simulink library "lib_Actuators"  (R2017a)
settings: Solver=VariableStepAuto  StartTime=0.0  StopTime=10.0  RelTol=1e-3
settings Model: Creator=Di Russo  LastModifiedBy=Vraj M

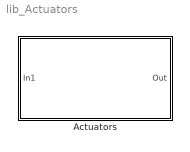
== system lib_Actuators ==
  Actuators : Subsystem

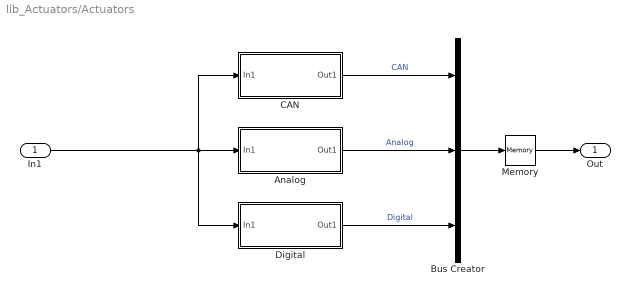
== system lib_Actuators/Actuators ==
  In1 : Inport
  Analog : Subsystem
  Bus Creator : BusCreator  Inputs=3
  CAN : Subsystem
  Digital : Subsystem
  Memory : Memory  InheritSampleTime=on
  Out : Outport
  wires:
  Memory/1 -> Out/1
  Analog/1(Out1) -> Bus Creator/2  "Analog"
  CAN/1(Out1) -> Bus Creator/1  "CAN"
  Digital/1(Out1) -> Bus Creator/3  "Digital"
  Bus Creator/1 -> Memory/1
  In1/1 -> Digital/1(In1), Analog/1(In1), CAN/1(In1)

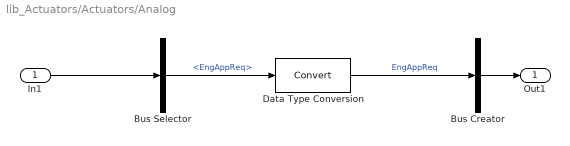
== system lib_Actuators/Actuators/Analog ==
  In1 : Inport
  Bus Creator : BusCreator  Inputs=1
  Bus Selector : BusSelector  OutputSignals=Controls.EngAppReq
  Data Type Conversion : DataTypeConversion
  Out1 : Outport
  wires:
  Data Type Conversion/1 -> Bus Creator/1  "EngAppReq"
  Bus Selector/1 -> Data Type Conversion/1  "<EngAppReq>"
  Bus Creator/1 -> Out1/1
  In1/1 -> Bus Selector/1

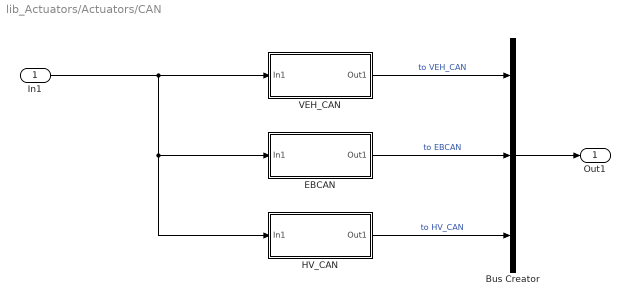
== system lib_Actuators/Actuators/CAN ==
  In1 : Inport
  Bus Creator : BusCreator  Inputs=3
  EBCAN : Subsystem
  HV_CAN : Subsystem
  VEH_CAN : Subsystem
  Out1 : Outport
  wires:
  In1/1 -> VEH_CAN/1(In1), EBCAN/1(In1), HV_CAN/1(In1)
  Bus Creator/1 -> Out1/1
  HV_CAN/1(Out1) -> Bus Creator/3  "to HV_CAN"
  EBCAN/1(Out1) -> Bus Creator/2  "to EBCAN"
  VEH_CAN/1(Out1) -> Bus Creator/1  "to VEH_CAN"

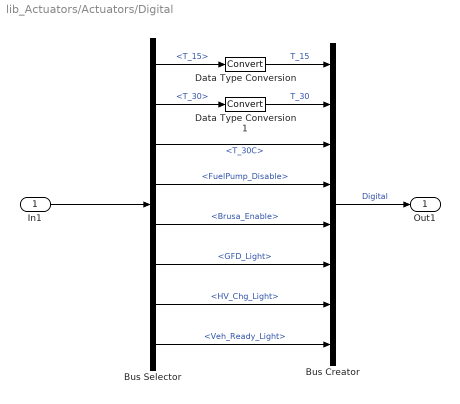
== system lib_Actuators/Actuators/Digital ==
  In1 : Inport
  Bus Creator : BusCreator  Inputs=8
  Bus Selector : BusSelector  OutputSignals=BMS_Digital.T_15,BMS_Digital.T_30,BMS_Digital.T_30C,Fuel_Pump_Control.Pump_Commands.FuelPump_Disable,OBC_Digital.Brusa_Enable,Axiomatic_CAN.GFD_Light,Axiomatic_CAN.HV_Chg_Light,Axiomatic_CAN.Veh_Ready_Light
  Data Type Conversion : DataTypeConversion
  Data Type Conversion1 : DataTypeConversion
  Out1 : Outport
  wires:
  Data Type Conversion1/1 -> Bus Creator/2  "T_30"
  Data Type Conversion/1 -> Bus Creator/1  "T_15"
  Bus Selector/8 -> Bus Creator/8  "<Veh_Ready_Light>"
  Bus Selector/7 -> Bus Creator/7  "<HV_Chg_Light>"
  Bus Selector/6 -> Bus Creator/6  "<GFD_Light>"
  Bus Selector/5 -> Bus Creator/5  "<Brusa_Enable>"
  Bus Selector/1 -> Data Type Conversion/1  "<T_15>"
  Bus Selector/2 -> Data Type Conversion1/1  "<T_30>"
  Bus Selector/3 -> Bus Creator/3  "<T_30C>"
  Bus Selector/4 -> Bus Creator/4  "<FuelPump_Disable>"
  Bus Creator/1 -> Out1/1  "Digital"
  In1/1 -> Bus Selector/1

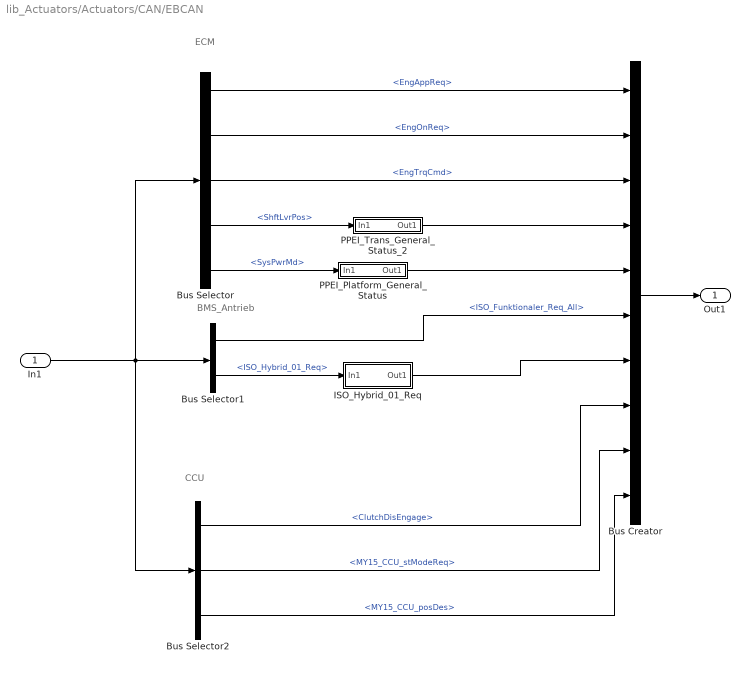
== system lib_Actuators/Actuators/CAN/EBCAN ==
  note: CCU
  note: ECM
  note: BMS_Antrieb
  In1 : Inport
  Bus Creator : BusCreator  Inputs=10
  Bus Selector : BusSelector  OutputSignals=Controls.EngAppReq,Controls.EngOnReq,Controls.EngTrqCmd,Controls.ShftLvrPos,Controls.SysPwrMd
  Bus Selector1 : BusSelector  OutputSignals=BMS_CAN.ISO_Funktionaler_Req_All,BMS_CAN.ISO_Hybrid_01_Req
  Bus Selector2 : BusSelector  OutputSignals=Controls.ClutchDisEngage,CCU_CAN.MY15_CCU_stModeReq,CCU_CAN.MY15_CCU_posDes
  ISO_Hybrid_01_Req : Subsystem
  PPEI_Platform_General_Status : Subsystem
  PPEI_Trans_General_Status_2 : Subsystem
  Out1 : Outport
  wires:
  Bus Selector2/1 -> Bus Creator/8  "<ClutchDisEngage>"
  Bus Selector2/3 -> Bus Creator/10  "<MY15_CCU_posDes>"
  Bus Selector2/2 -> Bus Creator/9  "<MY15_CCU_stModeReq>"
  In1/1 -> Bus Selector1/1, Bus Selector2/1, Bus Selector/1
  Bus Selector1/2 -> ISO_Hybrid_01_Req/1(In1)  "<ISO_Hybrid_01_Req>"
  ISO_Hybrid_01_Req/1(Out1) -> Bus Creator/7
  Bus Selector1/1 -> Bus Creator/6  "<ISO_Funktionaler_Req_All>"
  Bus Selector/1 -> Bus Creator/1  "<EngAppReq>"
  Bus Selector/2 -> Bus Creator/2  "<EngOnReq>"
  Bus Selector/3 -> Bus Creator/3  "<EngTrqCmd>"
  PPEI_Trans_General_Status_2/1(Out1) -> Bus Creator/4
  Bus Selector/5 -> PPEI_Platform_General_Status/1(In1)  "<SysPwrMd>"
  Bus Selector/4 -> PPEI_Trans_General_Status_2/1(In1)  "<ShftLvrPos>"
  PPEI_Platform_General_Status/1(Out1) -> Bus Creator/5
  Bus Creator/1 -> Out1/1

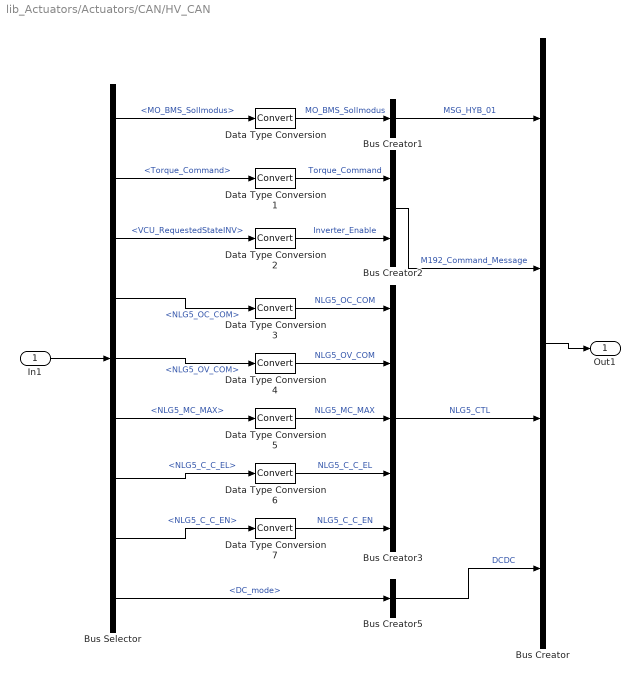
== system lib_Actuators/Actuators/CAN/HV_CAN ==
  In1 : Inport
  Bus Creator : BusCreator  Inputs=4
  Bus Creator1 : BusCreator  Inputs=1
  Bus Creator2 : BusCreator  Inputs=2
  Bus Creator3 : BusCreator  Inputs=5
  Bus Creator5 : BusCreator  Inputs=1
  Bus Selector : BusSelector  OutputSignals=BMS_CAN.MSG_HYB_01.MO_BMS_Sollmodus,Controls.Torque_Command,MCU_CAN.MCU_CAN.VCU_RequestedStateINV,OBC_CAN.NLG5_OC_COM,OBC_CAN.NLG5_OV_COM,OBC_CAN.NLG5_MC_MAX,OBC_CAN.NLG5_C_C_EL,OBC_CAN.NLG5_C_C_EN,MCU_CAN.DCDC_Out.DC_mode
  Data Type Conversion{,1..7} (8 alike) : DataTypeConversion
  Out1 : Outport
  wires:
  Bus Creator5/1 -> Bus Creator/4  "DCDC"
  Bus Selector/9 -> Bus Creator5/1  "<DC_mode>"
  Data Type Conversion7/1 -> Bus Creator3/5  "NLG5_C_C_EN"
  Data Type Conversion6/1 -> Bus Creator3/4  "NLG5_C_C_EL"
  Data Type Conversion5/1 -> Bus Creator3/3  "NLG5_MC_MAX"
  Data Type Conversion4/1 -> Bus Creator3/2  "NLG5_OV_COM"
  Data Type Conversion3/1 -> Bus Creator3/1  "NLG5_OC_COM"
  Bus Creator3/1 -> Bus Creator/3  "NLG5_CTL"
  Data Type Conversion2/1 -> Bus Creator2/2  "Inverter_Enable"
  Data Type Conversion1/1 -> Bus Creator2/1  "Torque_Command"
  Bus Selector/8 -> Data Type Conversion7/1  "<NLG5_C_C_EN>"
  Bus Selector/7 -> Data Type Conversion6/1  "<NLG5_C_C_EL>"
  Bus Selector/6 -> Data Type Conversion5/1  "<NLG5_MC_MAX>"
  Bus Selector/5 -> Data Type Conversion4/1  "<NLG5_OV_COM>"
  Bus Selector/4 -> Data Type Conversion3/1  "<NLG5_OC_COM>"
  Bus Creator2/1 -> Bus Creator/2  "M192_Command_Message"
  Bus Selector/3 -> Data Type Conversion2/1  "<VCU_RequestedStateINV>"
  Bus Selector/2 -> Data Type Conversion1/1  "<Torque_Command>"
  Bus Creator1/1 -> Bus Creator/1  "MSG_HYB_01"
  Data Type Conversion/1 -> Bus Creator1/1  "MO_BMS_Sollmodus"
  Bus Selector/1 -> Data Type Conversion/1  "<MO_BMS_Sollmodus>"
  In1/1 -> Bus Selector/1
  Bus Creator/1 -> Out1/1

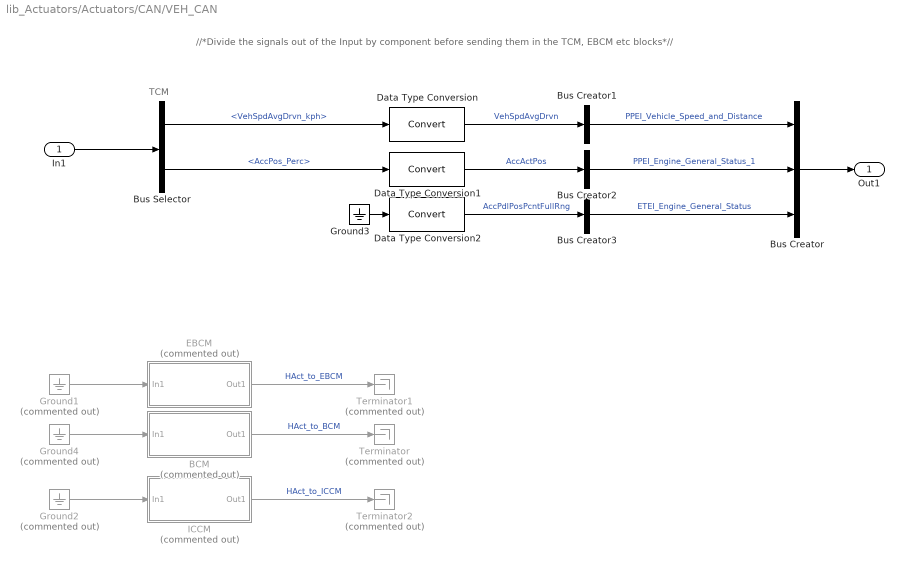
== system lib_Actuators/Actuators/CAN/VEH_CAN ==
  note: //*Divide the signals out of the Input by component before sending them in the TCM, EBCM etc blocks*//
  note: TCM
  In1 : Inport
  BCM : Subsystem  Commented=on
  Bus Creator : BusCreator  Inputs=3
  Bus Creator1 : BusCreator  Inputs=1
  Bus Creator2 : BusCreator  Inputs=1
  Bus Creator3 : BusCreator  Inputs=1
  Bus Selector : BusSelector  OutputSignals=Controls.VehSpdAvgDrvn_kph,Controls.AccPos_Perc
  Data Type Conversion : DataTypeConversion
  Data Type Conversion1 : DataTypeConversion
  Data Type Conversion2 : DataTypeConversion
  EBCM : Subsystem  Commented=on
  Ground1 : Ground  Commented=on
  Ground2 : Ground  Commented=on
  Ground3 : Ground
  Ground4 : Ground  Commented=on
  ICCM : Subsystem  Commented=on
  Terminator : Terminator  Commented=on
  Terminator1 : Terminator  Commented=on
  Terminator2 : Terminator  Commented=on
  Out1 : Outport
  wires:
  Ground4/1 -> BCM/1(In1)
  Ground3/1 -> Data Type Conversion2/1
  Data Type Conversion2/1 -> Bus Creator3/1  "AccPdlPosPcntFullRng"
  Bus Creator3/1 -> Bus Creator/3  "ETEI_Engine_General_Status"
  Bus Creator2/1 -> Bus Creator/2  "PPEI_Engine_General_Status_1"
  Data Type Conversion1/1 -> Bus Creator2/1  "AccActPos"
  Bus Creator1/1 -> Bus Creator/1  "PPEI_Vehicle_Speed_and_Distance"
  In1/1 -> Bus Selector/1
  Bus Selector/1 -> Data Type Conversion/1  "<VehSpdAvgDrvn_kph>"
  Bus Selector/2 -> Data Type Conversion1/1  "<AccPos_Perc>"
  Ground2/1 -> ICCM/1(In1)
  Ground1/1 -> EBCM/1(In1)
  Bus Creator/1 -> Out1/1
  Data Type Conversion/1 -> Bus Creator1/1  "VehSpdAvgDrvn"
  EBCM/1(Out1) -> Terminator1/1  "HAct_to_EBCM"
  BCM/1(Out1) -> Terminator/1  "HAct_to_BCM"
  ICCM/1(Out1) -> Terminator2/1  "HAct_to_ICCM"

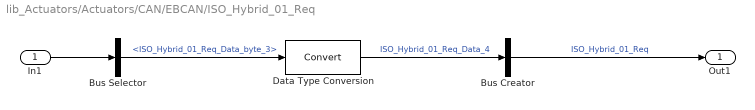
== system lib_Actuators/Actuators/CAN/EBCAN/ISO_Hybrid_01_Req ==
  In1 : Inport
  Bus Creator : BusCreator  Inputs=1
  Bus Selector : BusSelector  OutputSignals=ISO_Hybrid_01_Req_Data_byte_3
  Data Type Conversion : DataTypeConversion
  Out1 : Outport
  wires:
  Bus Selector/1 -> Data Type Conversion/1  "<ISO_Hybrid_01_Req_Data_byte_3>"
  Bus Creator/1 -> Out1/1  "ISO_Hybrid_01_Req"
  Data Type Conversion/1 -> Bus Creator/1  "ISO_Hybrid_01_Req_Data_4"
  In1/1 -> Bus Selector/1

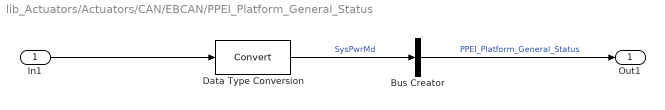
== system lib_Actuators/Actuators/CAN/EBCAN/PPEI_Platform_General_Status ==
  In1 : Inport
  Bus Creator : BusCreator  Inputs=1
  Data Type Conversion : DataTypeConversion
  Out1 : Outport
  wires:
  In1/1 -> Data Type Conversion/1
  Data Type Conversion/1 -> Bus Creator/1  "SysPwrMd"
  Bus Creator/1 -> Out1/1  "PPEI_Platform_General_Status"

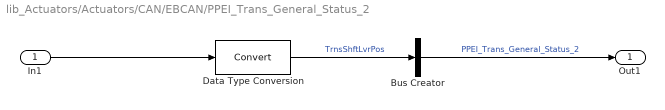
== system lib_Actuators/Actuators/CAN/EBCAN/PPEI_Trans_General_Status_2 ==
  In1 : Inport
  Bus Creator : BusCreator  Inputs=1
  Data Type Conversion : DataTypeConversion
  Out1 : Outport
  wires:
  Bus Creator/1 -> Out1/1  "PPEI_Trans_General_Status_2"
  Data Type Conversion/1 -> Bus Creator/1  "TrnsShftLvrPos"
  In1/1 -> Data Type Conversion/1

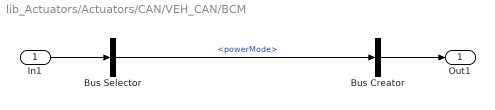
== system lib_Actuators/Actuators/CAN/VEH_CAN/BCM ==
  In1 : Inport
  Bus Creator : BusCreator  Inputs=1
  Bus Selector : BusSelector  OutputSignals=Controls.powerMode
  Out1 : Outport
  wires:
  Bus Creator/1 -> Out1/1
  Bus Selector/1 -> Bus Creator/1  "<powerMode>"
  In1/1 -> Bus Selector/1

== system lib_Actuators/Actuators/CAN/VEH_CAN/EBCM ==
  In1 : Inport
  Out1 : Outport
  wires:
  In1/1 -> Out1/1

== system lib_Actuators/Actuators/CAN/VEH_CAN/ICCM ==
  In1 : Inport
  Out1 : Outport
  wires:
  In1/1 -> Out1/1
